simulink model "buck_pi"  (R2018a)
settings: Solver=VariableStepAuto  StartTime=0.0  StopTime=0.09  RelTol=1e-3
undefined symbols (not defined in the file): sigbuilder_block
libraries: powerlib x15, simulink x2, powerlib_meascontrol x1
settings Model: Creator=KUNAL  LastModifiedBy=KUNAL

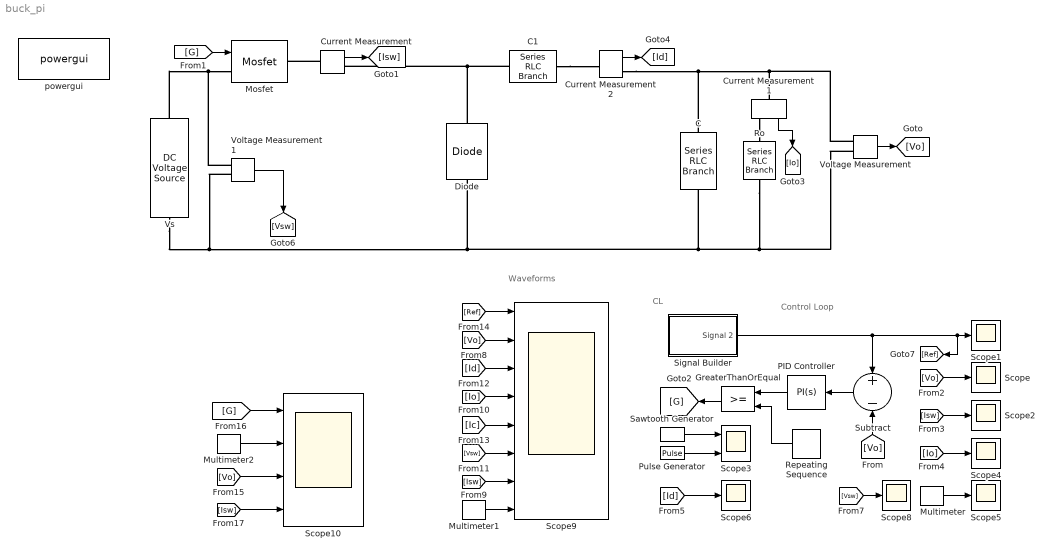
== system buck_pi ==
  note: Control Loop
  note: Waveforms
  note: CL
  C : powerlib/Elements/Series RLC Branch  LConnTagsString=__new0  RConnTagsString=__new0  BranchType=C  Resistance=0.01  Inductance=1e-3  SetiL0=off  InitialCurrent=0  Capacitance=0.25e-03  Setx0=off  InitialVoltage=0  Measurements=None
  C1 : powerlib/Elements/Series RLC Branch  LConnTagsString=__new0  RConnTagsString=__new0  BranchType=L  Resistance=0.01  Inductance=0.5  SetiL0=off  InitialCurrent=0  Capacitance=4.6e-05  Setx0=off  InitialVoltage=0  Measurements=None
  Current Measurement : powerlib/Measurements/Current Measurement  PhasorSimulation=off  OutputType=Complex  PSBequivalent=0
  Current Measurement1 : powerlib/Measurements/Current Measurement  PhasorSimulation=off  OutputType=Complex  PSBequivalent=0
  Current Measurement2 : powerlib/Measurements/Current Measurement  PhasorSimulation=off  OutputType=Complex  PSBequivalent=0
  Diode : powerlib/Power Electronics/Diode  Ron=0  Lon=0  Vf=0  IC=0  UseSnubber=off  Rs=inf  Cs=0  Measurements=off
  GreaterThanOrEqual : RelationalOperator  OutDataTypeStr=boolean  RndMeth=Simplest
  Mosfet : powerlib/Power Electronics/Mosfet  Ron=0.00000000000001  Lon=0  Rd=0  Vfd=0  IC=0  Rs=inf  Cs=0  Measurements=off
  Multimeter : powerlib/Measurements/Multimeter  PhasorSimulation=off  OutputType=Complex  sel=1  L=1  Gain=0  yselected={}  PSBOutputType=1  PSBequivalent=0  AxesSetting=[0,0.1,-100,100]  Display=0  SavedBlockNames=-11
  Multimeter1 : powerlib/Measurements/Multimeter  PhasorSimulation=off  OutputType=Complex  sel=1  L=1  Gain=0  yselected={}  PSBOutputType=1  PSBequivalent=0  AxesSetting=[0,0.1,-100,100]  Display=0  SavedBlockNames=-11
  Multimeter2 : powerlib/Measurements/Multimeter  PhasorSimulation=off  OutputType=Complex  sel=1  L=1  Gain=0  yselected={}  PSBOutputType=1  PSBequivalent=0  AxesSetting=[0,0.1,-100,100]  Display=0  SavedBlockNames=-11
  PID Controller : simulink/Continuous/PID Controller  Controller=PI  TimeDomain=Continuous-time  SampleTime=-1  IntegratorMethod=Forward Euler  FilterMethod=Forward Euler  Form=Parallel  UseFilter=on  ControllerParametersSource=internal  P=30  I=20  D=0.01  N=1000000000  InitialConditionSource=internal  InitialConditionForIntegrator=0  InitialConditionForFilter=0  ExternalReset=none  LimitOutput=off  UpperSaturationLimit=inf  LowerSaturationLimit=-inf  LinearizeAsGain=on  AntiWindupMode=none  Kb=1  TrackingMode=off  Kt=1  PParamMin=[]  PParamMax=[]  IParamMin=[]  IParamMax=[]  DParamMin=[]  DParamMax=[]  NParamMin=[]  NParamMax=[]  KbParamMin=[]  KbParamMax=[]  KtParamMin=[]  KtParamMax=[]  POutMin=[]  POutMax=[]  IOutMin=[]  IOutMax=[]  DOutMin=[]  DOutMax=[]  NOutMin=[]  NOutMax=[]  KbOutMin=[]  KbOutMax=[]  KtOutMin=[]  KtOutMax=[]  IntegratorOutMin=[]  IntegratorOutMax=[]  FilterOutMin=[]  FilterOutMax=[]  SumOutMin=[]  SumOutMax=[]  SumI1OutMin=[]  SumI1OutMax=[]  SumI2OutMin=[]  SumI2OutMax=[]  SumI3OutMin=[]  SumI3OutMax=[]  SumDOutMin=[]  SumDOutMax=[]  SaturationOutMin=[]  SaturationOutMax=[]  IntegratorContinuousStateAttributes=''  IntegratorStateMustResolveToSignalObject=off  IntegratorRTWStateStorageClass=Auto  FilterContinuousStateAttributes=''  FilterStateMustResolveToSignalObject=off  FilterRTWStateStorageClass=Auto  DifferentiatorICPrevScaledInput=0  DifferentiatorOutMin=[]  DifferentiatorOutMax=[]  FilterDiffOutCoefMin=[]  FilterDiffOutCoefMax=[]  SumDenOutMin=[]  SumDenOutMax=[]  SumNumOutMin=[]  SumNumOutMax=[]  ReciprocalOutMin=[]  ReciprocalOutMax=[]  DivideOutMin=[]  DivideOutMax=[]  TunerSelectOption=Transfer Function Based (PID Tuner App)
  Pulse Generator : DiscretePulseGenerator  PulseType=Time based  Period=1/100e3  PulseWidth=42.85714
  Repeating Sequence : simulink/Sources/Repeating Sequence  rep_seq_t=[0 1/100e3]  rep_seq_y=[0 1]
  Ro : powerlib/Elements/Series RLC Branch  LConnTagsString=__new0  RConnTagsString=__new0  BranchType=R  Resistance=50  Inductance=1e-3  SetiL0=off  InitialCurrent=0  Capacitance=1e-6  Setx0=off  InitialVoltage=0  Measurements=None
  Sawtooth Generator : powerlib_meascontrol/Pulse & Signal Generators/Sawtooth Generator  Freq=100e3  Phase=0  Ts=0
      settings: SourceProductName=Simscape Power Systems
  Scope{,1..2,4..6,8} (7 alike) : Scope
  Scope10 : Scope  NumInputPorts=4
  Scope3 : Scope  NumInputPorts=2
  Scope9 : Scope  NumInputPorts=8
  Signal Builder : Subsystem  Tag=STV Subsys  LoadFcn=sigbuilder_block('load');  StartFcn=sigbuilder_block('start');  StopFcn=sigbuilder_block('stop');  ClipboardFcn=sigbuilder_block('clipboard');  mask(Sigbuilder block){tuvar=[0:10]}
      mask help: Simulink:masks:SigbuilderBlock_MD
      mask init:
      | if ~strcmp(get_param(bdroot(gcbh),'SimulationStatus'),'stopped') tuvar = sigbuilder_block('maskInit'); end
      settings: CopyFcn=sigbuilder_block('copy');  DeleteFcn=sigbuilder_block('delete');  ModelCloseFcn=sigbuilder_block('modelClose');  PreSaveFcn=sigbuilder_block('preSave');  PauseFcn=sigbuilder_block('pause');  ContinueFcn=sigbuilder_block('continue');  NameChangeFcn=sigbuilder_block('namechange');  OpenFcn=sigbuilder_block('open',[6 30 1012.5 447.75 ]);  CloseFcn=sigbuilder_block('close');
      mask Display: plot(0, 0, 100, 100,[2, 2, 32, 32, 2], [68, 8, 8, 68, 68],[32, 2], [38, 38], [32, 19, 2],[53, 60, 44], [32, 17, 17, 2],[16, 16, 31, 31]);txt = getActiveGroup(gcbh);text(2, 100, txt,'verticalAlignment', 'top');
  Subtract : Sum  Inputs=+-
  Voltage Measurement : powerlib/Measurements/Voltage Measurement  PhasorSimulation=off  OutputType=Complex  PSBequivalent=0
  Voltage Measurement1 : powerlib/Measurements/Voltage Measurement  PhasorSimulation=off  OutputType=Complex  PSBequivalent=0
  Vs : powerlib/Electrical Sources/DC Voltage Source  Amplitude=220  Measurements=None
  powergui : powerlib/powergui  Priority=1  SimulationMode=Continuous  SampleTime=50e-6  frequency=60  Iterations=50  frequencyindice=0  Pbase=100e6  ErrMax=1e-4  UnitsV=kV  UnitsW=MW  buscounter=0  FunctionMessages=off  echomessages=off  EnableUseOfTLC=off  CurrentSourceSwitches=off  DisableSnubberDevices=off  DisableRonSwitches=off  DisableVfSwitches=off  DisplayEquations=off  SolverType=Tustin/Backward Euler (TBE)  Interpol=off  ExternalGateDelay=off  methode=off  Ts=100  x0status=blocks  SPID=on  SwTol=0  HookPort=off  RestoreLinks=warning  ResistiveCurrentMeasurement=off  Frange=[0:2:500]  Ylog=off  Xlog=on  ShowGrid=off  save=off  variable=ZData  structure=0  ZoomFFT=off  StartTime=0.0  cycles=1  DisplayStyle=1  fundamental=60  FreqAxis=off  MaxFrequency=1000  frequencyindicesteady=1  RmsSteady=1  display=off
  wires:
  Multimeter/1 -> Scope5/1
  [Vo] -> Subtract/2
  [G] -> Mosfet/1
  [Id] -> Scope6/1
  Voltage Measurement/1 -> [Vo]
  Multimeter2/1 -> Scope10/2
  [Isw] -> Scope9/7
  Multimeter1/1 -> Scope9/8
  [Vsw] -> Scope8/1
  [G] -> Scope10/1
  [Ref] -> Scope9/1
  [Isw] -> Scope2/1
  Pulse Generator/1 -> Scope3/2
  [Vo] -> Scope9/2
  [Io] -> Scope4/1
  Voltage Measurement1/1 -> [Vsw]
  [Vo] -> Scope/1
  [Ic] -> Scope9/5
  Current Measurement1/1 -> [Io]
  [Vsw] -> Scope9/6
  [Isw] -> Scope10/4
  Subtract/1 -> PID Controller/1
  [Vo] -> Scope10/3
  GreaterThanOrEqual/1 -> [G]
  Sawtooth Generator/1 -> Scope3/1
  PID Controller/1 -> GreaterThanOrEqual/1
  Repeating Sequence/1 -> GreaterThanOrEqual/2
  Current Measurement2/1 -> [Id]
  Signal Builder/1(Signal 2) -> Subtract/1, [Ref], Scope1/1
  [Id] -> Scope9/3
  [Io] -> Scope9/4
  Current Measurement/1 -> [Isw]
  connections:
  Voltage Measurement/LConn1 -- C/LConn1 -- Current Measurement2/RConn1 -- Current Measurement1/LConn1
  Current Measurement1/RConn1 -- Ro/LConn1
  Vs/RConn1 -- Voltage Measurement1/LConn1 -- Mosfet/LConn1
  C1/RConn1 -- Diode/RConn1 -- Current Measurement/RConn1
  Vs/LConn1 -- Voltage Measurement1/LConn2 -- Voltage Measurement/LConn2 -- Ro/RConn1 -- C/RConn1 -- Diode/LConn1
  C1/LConn1 -- Current Measurement2/LConn1
  Current Measurement/LConn1 -- Mosfet/RConn1

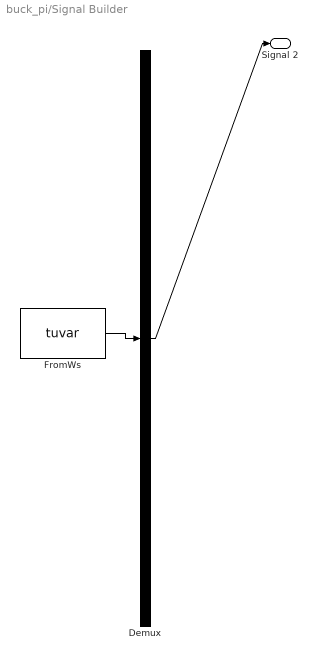
== system buck_pi/Signal Builder ==
  Demux : Demux  Tag=STV Demux  Outputs=1
  FromWs : FromWorkspace  Tag=STV FromWs  VariableName=tuvar  SampleTime=0
      SigBuilderData=|
      | common.afterFinalStr = 'Extrapolate'
      | common.sampleTime = 0
      | dataSet.timeRange = [0 0.09]
      | dataSet.name = 'Group 1'
      | sbobj.Groups.Name = 'Group 1'
      | sbobj.Groups.Signals.Name = 'Signal 2'
      | sbobj.Groups.Signals.XData = [0 0.09]
      | sbobj.Groups.Signals.YData = [110 110]
      | sbobj.Groups.TimeRange = [0 0.09]
  Signal 2 : Outport  Tag=STV Outport
  wires:
  FromWs/1 -> Demux/1
  Demux/1 -> Signal 2/1
